simulink model "untitled"  (R2025b)
settings: Solver=FixedStepAuto  StartTime=0.0  StopTime=10  FixedStep=0.05  RelTol=1e-3
settings Model: Creator=Dell  LastModifiedBy=Dell

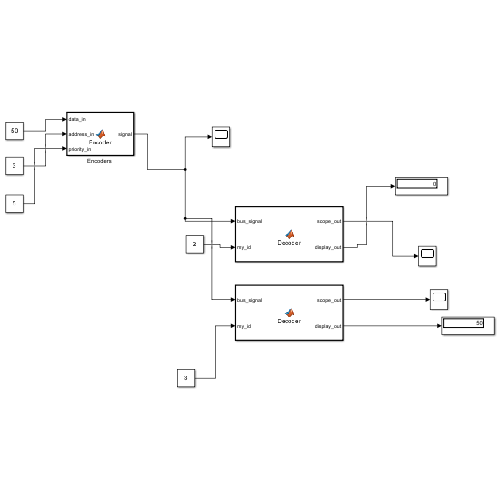
[thumbnail: Simulink's stored preview of the top-level diagram]
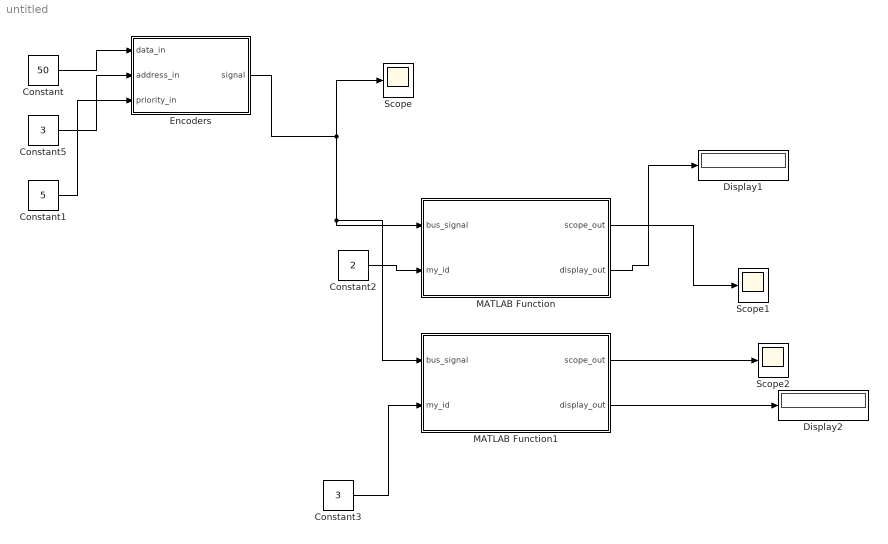
== system untitled ==
  Constant : Constant  Value=50
  Constant1 : Constant  Value=5
  Constant2 : Constant  Value=2
  Constant3 : Constant  Value=3
  Constant5 : Constant  Value=3
  Display1 : Display
  Display2 : Display
  "Encoders " : MATLAB Function  TreatAsAtomicUnit=on
  MATLAB Function : MATLAB Function  TreatAsAtomicUnit=on
  MATLAB Function1 : MATLAB Function  TreatAsAtomicUnit=on
  Scope : Scope
      settings: SampleTime=0.05  TimeSpan=4.1  ActiveDisplayYMinimum=-0.62499999999999989  ActiveDisplayYMaximum=5.625  DataLoggingVariableName=ScopeData2  DataLoggingSaveFormat=Array
  Scope1 : Scope
      settings: SampleTime=0.05  TimeSpan=4.1  ActiveDisplayYMinimum=-0.62499999999999989  ActiveDisplayYMaximum=5.625  DataLoggingSaveFormat=Array
  Scope2 : Scope
      settings: SampleTime=0.05  TimeSpan=4.1  ActiveDisplayYMinimum=-0.62499999999999989  ActiveDisplayYMaximum=5.625  DataLoggingSaveFormat=Array
  wires:
  Constant/1 -> "Encoders "/1(data_in)
  Constant5/1 -> "Encoders "/2(address_in)
  Constant1/1 -> "Encoders "/3(priority_in)
  Constant2/1 -> MATLAB Function/2(my_id)
  MATLAB Function/1(scope_out) -> Scope1/1
  MATLAB Function/2(display_out) -> Display1/1
  MATLAB Function1/2(display_out) -> Display2/1
  Constant3/1 -> MATLAB Function1/2(my_id)
  MATLAB Function1/1(scope_out) -> Scope2/1
  "Encoders "/1(signal) -> Scope/1, MATLAB Function1/1(bus_signal), MATLAB Function/1(bus_signal)

== matlab function untitled/MATLAB Function ==
  settings: updateMethod=DISCRETE  sampleTime=0.05
  data: scope_out output; bus_signal input; my_id input; display_out output
function [scope_out, display_out] = Decoder(bus_signal, my_id)
    % Persistent variables bit timing aur data store karne ke liye
    persistent state bit_count addr_buffer data_buffer result;
    
    if isempty(state)
        state = 0; % 0: Wait Start, 1: Skip Prio, 2: Check ID, 3: Pass & Convert
        bit_count = 0;
        addr_buffer = zeros(1,8);
        data_buffer = zeros(1,8);
        result = 0;
    end
    
    % Direct Voltage check (5V = High, 0V = Low)
    is_high = (bus_signal == 5); 
    
    % Default values
    scope_out = 0;
    display_out = result; % Display pe purana result dikhta rahega jab tak naya na aaye

    switch state
        case 0 % 1. WAIT FOR START BIT (5V)
            if is_high
                state = 1; 
                bit_count = 0;
            end
            
        case 1 % 2. SKIP HEADER + PRIORITY (10 BITS TOTAL)
            bit_count = bit_count + 1;
            if bit_count >= 10
                state = 2;
                bit_count = 0;
                addr_buffer = zeros(1,8);
            end
            
        case 2 % 3. CHECK ADDRESS VS DECODER ID
            bit_count = bit_count + 1;
            if bit_count <= 8
                addr_buffer(bit_count) = is_high;
            end
            if bit_count == 8
                received_id = sum(addr_buffer .* 2.^(7:-1:0));
                if received_id == my_id
                    state = 3; % ID Match: Gate Open
                    bit_count = 0;
                    data_buffer = zeros(1,8); % Data buffer reset
                else
                    state = 0; % Mismatch: Shut down for this cycle
                end
            end
            
        case 3 % 4. PASS SIGNAL TO SCOPE & CONVERT DATA TO DECIMAL
            bit_count = bit_count + 1;
            scope_out = bus_signal; % Scope pe wahi 5V pulses dikhayega
            
            % Data bits (16-bit doubled) ko wapis 8-bit decimal mein convert karna
            % Shuruat ke 20-bit gap ko skip karke data collect karna
            if bit_count > 20 
                data_tick = bit_count - 20;
                if data_tick <= 16 && mod(data_tick, 2) == 0
                    % Har 2nd bit (doubled) ko buffer mein store karna
                    data_buffer(data_tick/2) = is_high;
                end
            end
            
            % Jab pura frame khatam ho jaye (82 bits total) toh result update kar
            if bit_count >= 62
                result = double(sum(data_buffer .* 2.^(7:-1:0)));
                state = 0; % Reset for next cycle
            end
    end
end

== matlab function untitled/Encoders  ==
  settings: updateMethod=DISCRETE  sampleTime=0.05
  data: data_in input; signal output; address_in input; priority_in input
function signal = Encoder(data_in, address_in, priority_in)
    % Persistent variables allow the block to maintain its position in the frame
    persistent full_frame frame_index;
    
    % Initialization: This runs once to package your data into the protocol frame
    if isempty(frame_index)
        frame_index = 1;
        
        % 1. Convert decimal inputs to binary vectors (8-bit width)
        data_bits = bitget(uint8(data_in), 8:-1:1);
        addr_bits = bitget(uint8(address_in), 8:-1:1);
        prio_bits = bitget(uint8(priority_in), 8:-1:1);
        
        % 2. 16-bit Payload (Double Data Logic)
        % Sends two identical bits for every 1 bit of data for accuracy
        payload = reshape([data_bits; data_bits], 1, []);
        
        % 3. Assemble Frame with 0-Logic Delimiters
        % Start bit (1) followed by Process Start/Gap bit (0)
        header = [1, 0];
        
        % Priority (8-bit) followed by a Delimiter (0)
        prio_block = [double(prio_bits), 0];
        
        % Address (8-bit) followed by a Delimiter (0) - This is the "Data Starting Bit"
        addr_block = [double(addr_bits), 0];
        
        % Data Starting Gap (20 bits of logic 0)
        data_start_gap = zeros(1, 20);
        
        % Payload (16-bit doubled data)
        data_block = double(payload);
        
        % Post-data bits (20 bits of logic 0 for turnaround/feedback)
        data_end_gap = zeros(1, 20);
        
        % Acknowledgement (0, 1) and Stop bits (0, 0)
        tail = [0, 1, 0, 0];
        
        % 4. Combine all logic into the final sequence
        logic_sequence = [header, prio_block, addr_block, data_start_gap, data_block, data_end_gap, tail];
        
        % 5. Convert to Physical Voltage (+5V for Logic 1)
        full_frame = logic_sequence * 5; 
    end
    
    % Output exactly one voltage level per simulation time step
    signal = full_frame(frame_index);
    
    % Sequential index management
    if frame_index < length(full_frame)
        frame_index = frame_index + 1;
    else
        % Reset to 1 to loop the sequence for continuous observation on the Scope
        frame_index = 1; 
    end
end

== matlab function untitled/MATLAB Function1 ==
  settings: updateMethod=DISCRETE  sampleTime=0.05
  data: scope_out output; bus_signal input; my_id input; display_out output
function [scope_out, display_out] = Decoder(bus_signal, my_id)
    % Persistent variables bit timing aur data store karne ke liye
    persistent state bit_count addr_buffer data_buffer result;
    
    if isempty(state)
        state = 0; % 0: Wait Start, 1: Skip Prio, 2: Check ID, 3: Pass & Convert
        bit_count = 0;
        addr_buffer = zeros(1,8);
        data_buffer = zeros(1,8);
        result = 0;
    end
    
    % Direct Voltage check (5V = High, 0V = Low)
    is_high = (bus_signal == 5); 
    
    % Default values
    scope_out = 0;
    display_out = result; % Display pe purana result dikhta rahega jab tak naya na aaye

    switch state
        case 0 % 1. WAIT FOR START BIT (5V)
            if is_high
                state = 1; 
                bit_count = 0;
            end
            
        case 1 % 2. SKIP HEADER + PRIORITY (10 BITS TOTAL)
            bit_count = bit_count + 1;
            if bit_count >= 10
                state = 2;
                bit_count = 0;
                addr_buffer = zeros(1,8);
            end
            
        case 2 % 3. CHECK ADDRESS VS DECODER ID
            bit_count = bit_count + 1;
            if bit_count <= 8
                addr_buffer(bit_count) = is_high;
            end
            if bit_count == 8
                received_id = sum(addr_buffer .* 2.^(7:-1:0));
                if received_id == my_id
                    state = 3; % ID Match: Gate Open
                    bit_count = 0;
                    data_buffer = zeros(1,8); % Data buffer reset
                else
                    state = 0; % Mismatch: Shut down for this cycle
                end
            end
            
        case 3 % 4. PASS SIGNAL TO SCOPE & CONVERT DATA TO DECIMAL
            bit_count = bit_count + 1;
            scope_out = bus_signal; % Scope pe wahi 5V pulses dikhayega
            
            % Data bits (16-bit doubled) ko wapis 8-bit decimal mein convert karna
            % Shuruat ke 20-bit gap ko skip karke data collect karna
            if bit_count > 20 
                data_tick = bit_count - 20;
                if data_tick <= 16 && mod(data_tick, 2) == 0
                    % Har 2nd bit (doubled) ko buffer mein store karna
                    data_buffer(data_tick/2) = is_high;
                end
            end
            
            % Jab pura frame khatam ho jaye (82 bits total) toh result update kar
            if bit_count >= 62
                result = double(sum(data_buffer .* 2.^(7:-1:0)));
                state = 0; % Reset for next cycle
            end
    end
end
